simulink model "Q6"  (R2014b)
settings: Solver=ode45  StartTime=0.0  StopTime=50  RelTol=1e-3
undefined symbols (not defined in the file or in its folder): sigbuilder_block
libraries: simulink x1
settings Model: Creator=Ashish  LastModifiedBy=Ashish

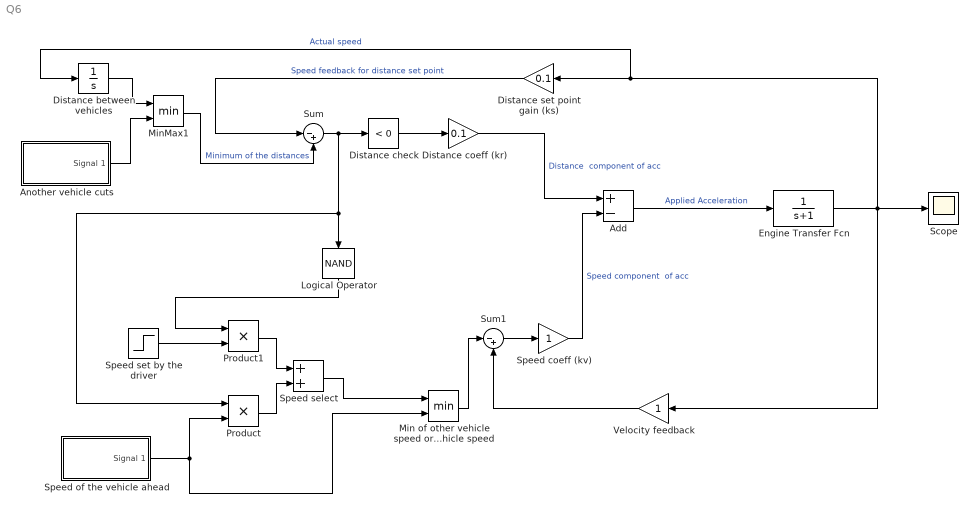
== system Q6 ==
  Add : Sum  Inputs=+-
  Another vehicle cuts : Subsystem  Tag=STV Subsys  LoadFcn=sigbuilder_block('load');  StartFcn=sigbuilder_block('start');  StopFcn=sigbuilder_block('stop');  ClipboardFcn=sigbuilder_block('clipboard');  mask(Sigbuilder block){}
      mask help: Simulink:masks:SigbuilderBlock_MD
      mask init:
      | if ~strcmp(get_param(bdroot(gcbh),'SimulationStatus'),'stopped') tuvar = sigbuilder_block('maskInit'); end
      settings: CopyFcn=sigbuilder_block('copy');  DeleteFcn=sigbuilder_block('delete');  ModelCloseFcn=sigbuilder_block('modelClose');  PreSaveFcn=sigbuilder_block('preSave');  PauseFcn=sigbuilder_block('pause');  ContinueFcn=sigbuilder_block('continue');  NameChangeFcn=sigbuilder_block('namechange');  OpenFcn=sigbuilder_block('open',[437.6 199.2 550.4 400 ]);  CloseFcn=sigbuilder_block('close');
      mask Display: plot(0, 0, 100, 100,[2, 2, 32, 32, 2], [68, 8, 8, 68, 68],[32, 2], [38, 38], [32, 19, 2],[53, 60, 44], [32, 17, 17, 2],[16, 16, 31, 31]);txt = getActiveGroup(gcbh);text(2, 100, txt,'verticalAlignment', 'top');
  Distance check : simulink/Logic and Bit Operations/Compare To Zero  relop=<  OutDataTypeStr=boolean
  Distance coeff (kr) : Gain  Gain=0.1
  Distance between vehicles : Integrator  InitialCondition=10
  Distance set point gain (ks) : Gain  Gain=0.1
  Engine Transfer Fcn : TransferFcn  Numerator=1  Denominator=[1 1]
  Logical Operator : Logic  Operator=NAND  Inputs=1  AllPortsSameDT=off  OutDataTypeStr=boolean
  Min of other vehicle speed or host vehicle speed : MinMax  Inputs=2
  MinMax1 : MinMax  Inputs=2
  Product : Product
  Product1 : Product
  Scope : Scope
      settings: YMin=79.83  YMax=79.92
  Speed select : Sum
  Speed coeff (kv) : Gain
  Speed of the vehicle ahead : Subsystem  Tag=STV Subsys  LoadFcn=sigbuilder_block('load');  StartFcn=sigbuilder_block('start');  StopFcn=sigbuilder_block('stop');  ClipboardFcn=sigbuilder_block('clipboard');  mask(Sigbuilder block){}
      mask help: Simulink:masks:SigbuilderBlock_MD
      mask init:
      | if ~strcmp(get_param(bdroot(gcbh),'SimulationStatus'),'stopped') tuvar = sigbuilder_block('maskInit'); end
      settings: CopyFcn=sigbuilder_block('copy');  DeleteFcn=sigbuilder_block('delete');  ModelCloseFcn=sigbuilder_block('modelClose');  PreSaveFcn=sigbuilder_block('preSave');  PauseFcn=sigbuilder_block('pause');  ContinueFcn=sigbuilder_block('continue');  NameChangeFcn=sigbuilder_block('namechange');  OpenFcn=sigbuilder_block('open',[437.6 199.2 550.4 400 ]);  CloseFcn=sigbuilder_block('close');
      mask Display: plot(0, 0, 100, 100,[2, 2, 32, 32, 2], [68, 8, 8, 68, 68],[32, 2], [38, 38], [32, 19, 2],[53, 60, 44], [32, 17, 17, 2],[16, 16, 31, 31]);txt = getActiveGroup(gcbh);text(2, 100, txt,'verticalAlignment', 'top');
  Speed set by the driver : Step  Time=5  Before=50  After=70  SampleTime=0
  Sum : Sum  Inputs=|-+
  Sum1 : Sum  Inputs=|-+
  Velocity feedback : Gain
  wires:
  Sum/1 -> Distance check/1, Product/1, Logical Operator/1
  Min of other vehicle speed or host vehicle speed/1 -> Sum1/1
  Sum1/1 -> Speed coeff (kv)/1
  Add/1 -> Engine Transfer Fcn/1  "Applied Acceleration"
  Speed coeff (kv)/1 -> Add/2  "Speed component  of acc"
  Engine Transfer Fcn/1 -> Velocity feedback/1, Distance between vehicles/1, Distance set point gain (ks)/1, Scope/1  "Actual speed"
  Distance set point gain (ks)/1 -> Sum/1  "Speed feedback for distance set point"
  Velocity feedback/1 -> Sum1/2
  Distance coeff (kr)/1 -> Add/1  "Distance  component of acc"
  Distance check/1 -> Distance coeff (kr)/1
  Speed of the vehicle ahead/1(Signal 1) -> Min of other vehicle speed or host vehicle speed/2, Product/2
  Speed set by the driver/1 -> Product1/2
  Logical Operator/1 -> Product1/1
  Product1/1 -> Speed select/1
  Product/1 -> Speed select/2
  Speed select/1 -> Min of other vehicle speed or host vehicle speed/1
  Distance between vehicles/1 -> MinMax1/1
  Another vehicle cuts/1(Signal 1) -> MinMax1/2
  MinMax1/1 -> Sum/2  "Minimum of the distances"

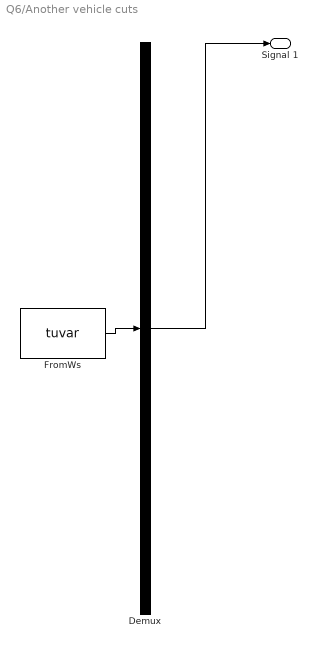
== system Q6/Another vehicle cuts ==
  Demux : Demux  Tag=STV Demux  Outputs=1
  FromWs : FromWorkspace  Tag=STV FromWs  VariableName=tuvar  SampleTime=0
      SigBuilderData=|
      | common.afterFinalStr = 'Extrapolate'
      | common.sampleTime = 0
      | dataSet.timeRange = [0 100]
      | dataSet.name = 'Group 1'
      | sbobj.Groups.Name = 'Group 1'
      | sbobj.Groups.Signals.Name = 'Signal 1'
      | sbobj.Groups.Signals.XData = [0 10 10 20 20 100]
      | sbobj.Groups.Signals.YData = [5 5 10 10 7 7]
      | sbobj.Groups.TimeRange = [0 100]
  Signal 1 : Outport  Tag=STV Outport
  wires:
  Demux/1 -> Signal 1/1
  FromWs/1 -> Demux/1

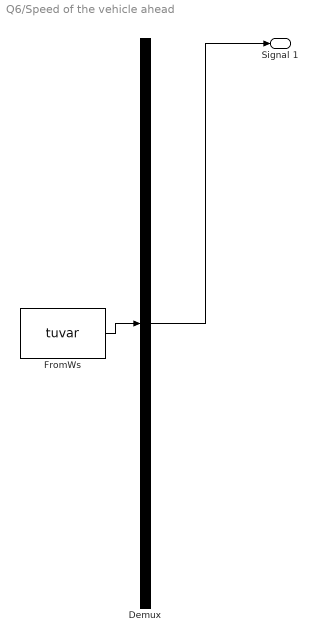
== system Q6/Speed of the vehicle ahead ==
  Demux : Demux  Tag=STV Demux  Outputs=1
  FromWs : FromWorkspace  Tag=STV FromWs  VariableName=tuvar  SampleTime=0
      SigBuilderData=|
      | common.afterFinalStr = 'Extrapolate'
      | common.sampleTime = 0
      | dataSet.timeRange = [0 100]
      | dataSet.name = 'Group 1'
      | sbobj.Groups.Name = 'Group 1'
      | sbobj.Groups.Signals.Name = 'Signal 1'
      | sbobj.Groups.Signals.XData = [0 10 10 20 20 100]
      | sbobj.Groups.Signals.YData = [60 60 40 40 80 80]
      | sbobj.Groups.TimeRange = [0 100]
  Signal 1 : Outport  Tag=STV Outport
  wires:
  Demux/1 -> Signal 1/1
  FromWs/1 -> Demux/1
